simulink model "parte3_DC1A"  (R2019b)
settings: Solver=VariableStepAuto  StartTime=0.0  StopTime=10  RelTol=1e-3
settings Model: Creator=Admon  LastModifiedBy=cjuar
settings DataIOCC: ReturnWorkspaceOutputs=off
settings DebuggingCC: ArithmeticOperatorsInVariantConditions=warning
settings SFSimCC: SimUseLocalCustomCode=off  CustomCodeUndefinedFunction=UseInterfaceOnly
settings RTWCC: RTWUseLocalCustomCode=off

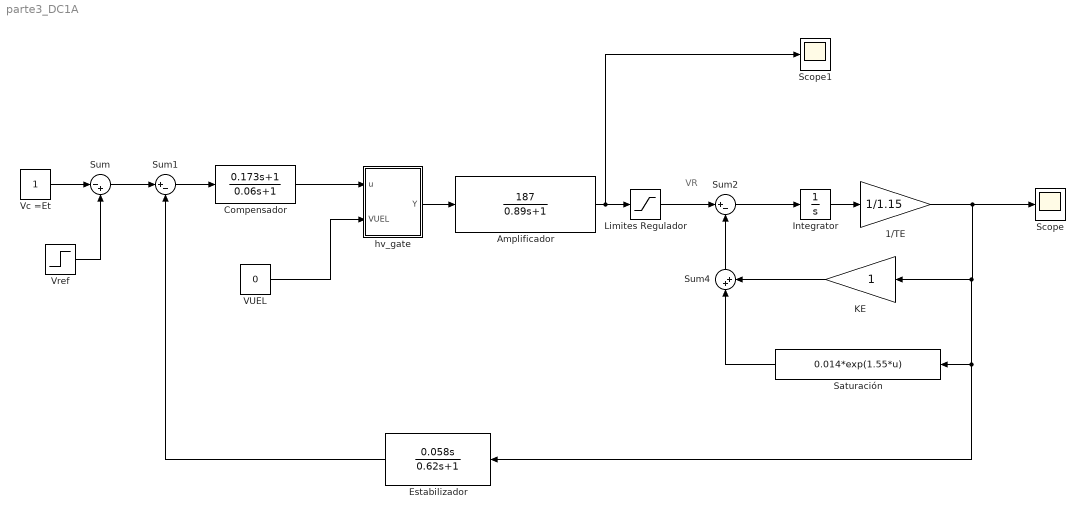
== system parte3_DC1A ==
  note: VR
  1/TE : Gain  Gain=1/1.15
  Amplificador : TransferFcn  Numerator=[187]  Denominator=[0.89 1]
  Compensador : TransferFcn  Numerator=[0.173 1]  Denominator=[0.06 1]
  Estabilizador : TransferFcn  Numerator=[0.058 0]  Denominator=[0.62 1]
  Integrator : Integrator
  KE : Gain
  Limites Regulador : Saturate  UpperLimit=1.7  LowerLimit=-1.7
  Saturación : Fcn  Expr=0.014*exp(1.55*u)
  Scope : Scope
  Scope1 : Scope
  Sum : Sum  Inputs=|-+
  Sum1 : Sum  Inputs=|+-
  Sum2 : Sum  Inputs=|+-
  Sum4 : Sum  Inputs=|++
  VUEL : Constant  Value=0
  Vc =Et : Constant
  Vref : Step  Before=1  SampleTime=0
  hv_gate : Subsystem
  wires:
  Sum/1 -> Sum1/1
  Sum1/1 -> Compensador/1
  Vc =Et/1 -> Sum/1
  Vref/1 -> Sum/2
  Estabilizador/1 -> Sum1/2
  hv_gate/1(Y) -> Amplificador/1
  Compensador/1 -> hv_gate/1(u)
  VUEL/1 -> hv_gate/2(VUEL)
  Amplificador/1 -> Scope1/1, Limites Regulador/1
  Limites Regulador/1 -> Sum2/1
  Sum2/1 -> Integrator/1
  Integrator/1 -> 1/TE/1
  1/TE/1 -> Estabilizador/1, Saturación/1, KE/1, Scope/1
  Sum4/1 -> Sum2/2
  KE/1 -> Sum4/2
  Saturación/1 -> Sum4/1

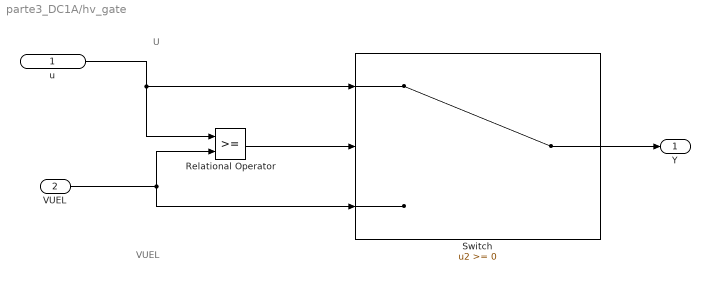
== system parte3_DC1A/hv_gate ==
  note: VUEL
  note: U
  u : Inport
  VUEL : Inport  Port=2
  Relational Operator : RelationalOperator  OutDataTypeStr=boolean  RndMeth=Simplest
  Switch : Switch
  Y : Outport  VectorParamsAs1DForOutWhenUnconnected=off
  wires:
  Relational Operator/1 -> Switch/2
  VUEL/1 -> Switch/3, Relational Operator/2
  u/1 -> Relational Operator/1, Switch/1
  Switch/1 -> Y/1
